simulink model "mnist_cnn_adam_figure"  (R2017b)
settings: Solver=FixedStepDiscrete  StartTime=0.0  StopTime=Inf  FixedStep=1  RelTol=1e-3
model workspace (MATLAB code in the model file):
  | filtersize1 = 5;
  | filtersize2 = 5;
  | features1 = 16;
  | features2 = 16;
  | densesize = 64;
  | classes = 10;
  | batchsize = 64;
libraries: ad_blocks x24
settings Model: PauseTimes=2  SnapshotBufferSize=2  SnapshotInterval=1  Creator=percro2  LastModifiedBy=eruffaldi
settings DataIOCC: ReturnWorkspaceOutputs=on
settings OptimizationCC: DefaultParameterBehavior=Inlined  InlineInvariantSignals=on  SimCompilerOptimization=on
settings RTWCC: GenerateReport=on  Toolchain=Clang v3.1 | gmake (64-bit Mac)  BuildConfiguration=Specify  LaunchReport=on
settings CodeAppCC: StateflowObjectComments=on  MATLABSourceComments=on
settings GRTTargetCC: CodeReplacementLibrary=GNU C99 extensions

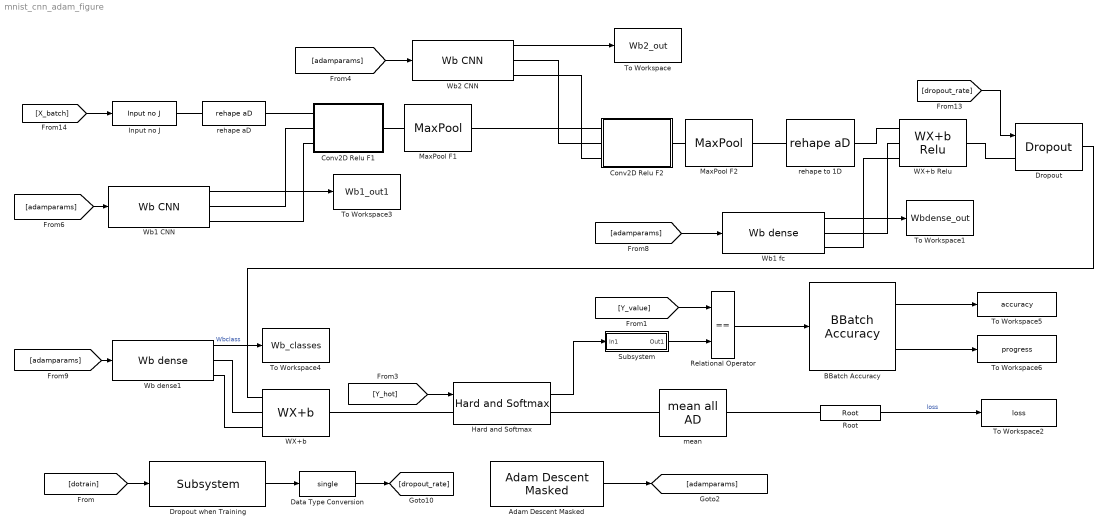
== system mnist_cnn_adam_figure ==
  Adam Descent Masked : ad_blocks/Adam Descent Masked  learningrate=1e-4  beta1=0.9  beta2=0.9999  epsilon=1e-8  adam=on
  BBatch Accuracy : ad_blocks/BBatch Accuracy
  Conv2D Relu F1 : Subsystem
  Conv2D Relu F2 : Subsystem
  Data Type Conversion : DataTypeConversion  OutDataTypeStr=single
  Dropout : ad_blocks/Dropout
  Dropout when Training : ad_blocks/Subsystem  dropout_rate=0.8
  Hard and Softmax : ad_blocks/Hard and Softmax
  Input no J : ad_blocks/Input no J  SystemSampleTime=-1
  MaxPool F1 : ad_blocks/MaxPool  stride=[1,2,2,1]  ksize=[1,2,2,1]  padding=-1
  MaxPool F2 : ad_blocks/MaxPool  stride=[1,2,2,1]  ksize=[1,2,2,1]  padding=-1
  Relational Operator : RelationalOperator  Operator===  OutDataTypeStr=boolean  RndMeth=Simplest
  Root : ad_blocks/Root  Description=Top level AD block: gets the incoming value, pushes the scalar 1 gradient  SystemSampleTime=-1
  Subsystem : Subsystem
  To Workspace : ToWorkspace  VariableName=Wb2_out  SaveFormat=Timeseries  SampleTime=-1
      settings: MaxDataPoints=1
  To Workspace1 : ToWorkspace  VariableName=Wbdense_out  SaveFormat=Timeseries  SampleTime=-1
      settings: MaxDataPoints=1
  To Workspace2 : ToWorkspace  VariableName=loss  SaveFormat=Timeseries  SampleTime=-1
      settings: MaxDataPoints=1
  To Workspace3 : ToWorkspace  VariableName=Wb1_out1  SaveFormat=Timeseries  SampleTime=-1
      settings: MaxDataPoints=1
  To Workspace4 : ToWorkspace  VariableName=Wb_classes  SaveFormat=Timeseries  SampleTime=-1
      settings: MaxDataPoints=1
  To Workspace5 : ToWorkspace  VariableName=accuracy  SaveFormat=Timeseries  SampleTime=-1
      settings: MaxDataPoints=1
  To Workspace6 : ToWorkspace  VariableName=progress  SaveFormat=Timeseries  SampleTime=-1
      settings: MaxDataPoints=1
  "WX+b " : ad_blocks/WX+b 
  WX+b Relu : ad_blocks/WX+b Relu
  Wb dense1 : ad_blocks/Wb dense  wshape=[densesize,classes]
  Wb1 CNN : ad_blocks/Wb CNN  K=filtersize1  Fi=1  Fo=features1
  Wb1 fc : ad_blocks/Wb dense  wshape=[7*7*features2,densesize]
  Wb2 CNN : ad_blocks/Wb CNN  K=filtersize2  Fi=features1  Fo=features2
  mean : ad_blocks/mean all AD
  rehape aD : ad_blocks/rehape aD  shape=[-1,28,28]
  rehape to 1D : ad_blocks/rehape aD  shape=[-1,-1]
  wires:
  [Y_value] -> Relational Operator/1
  Wb2 CNN/1 -> To Workspace/1
  [adamparams] -> Wb2 CNN/1
  [adamparams] -> Wb1 CNN/1
  Wb1 CNN/1 -> To Workspace3/1
  Wb1 fc/1 -> To Workspace1/1
  [adamparams] -> Wb1 fc/1
  Wb dense1/1 -> To Workspace4/1  "Wbclass"
  [adamparams] -> Wb dense1/1
  Relational Operator/1 -> BBatch Accuracy/2
  Dropout when Training/1 -> Data Type Conversion/1
  [dropout_rate] -> Dropout/1
  [dotrain] -> Dropout when Training/1
  Data Type Conversion/1 -> [dropout_rate]
  [X_batch] -> Input no J/1
  BBatch Accuracy/1 -> To Workspace5/1
  Root/1 -> To Workspace2/1  "loss"
  [Y_hot] -> Hard and Softmax/1
  Hard and Softmax/1 -> Subsystem/1(In1)
  Adam Descent Masked/1 -> [adamparams]
  Subsystem/1(Out1) -> Relational Operator/2
  BBatch Accuracy/2 -> To Workspace6/1
  connections:
  rehape aD/LConn1 -- Input no J/RConn1
  mean/RConn1 -- Root/LConn1
  MaxPool F2/LConn1 -- Conv2D Relu F2/RConn1
  rehape to 1D/LConn1 -- MaxPool F2/RConn1
  Dropout/LConn1 -- WX+b Relu/RConn1
  "WX+b "/LConn1 -- Dropout/RConn1
  "WX+b "/LConn2 -- Wb dense1/RConn1
  "WX+b "/LConn3 -- Wb dense1/RConn2
  Wb1 CNN/RConn2 -- Conv2D Relu F1/LConn3
  rehape to 1D/RConn1 -- WX+b Relu/LConn1
  Wb2 CNN/RConn1 -- Conv2D Relu F2/LConn2
  Wb2 CNN/RConn2 -- Conv2D Relu F2/LConn3
  Wb1 fc/RConn1 -- WX+b Relu/LConn2
  Wb1 fc/RConn2 -- WX+b Relu/LConn3
  Hard and Softmax/LConn1 -- "WX+b "/RConn1
  Hard and Softmax/RConn1 -- mean/LConn1
  MaxPool F1/RConn1 -- Conv2D Relu F2/LConn1
  Conv2D Relu F1/RConn1 -- MaxPool F1/LConn1
  rehape aD/RConn1 -- Conv2D Relu F1/LConn1
  Wb1 CNN/RConn1 -- Conv2D Relu F1/LConn2

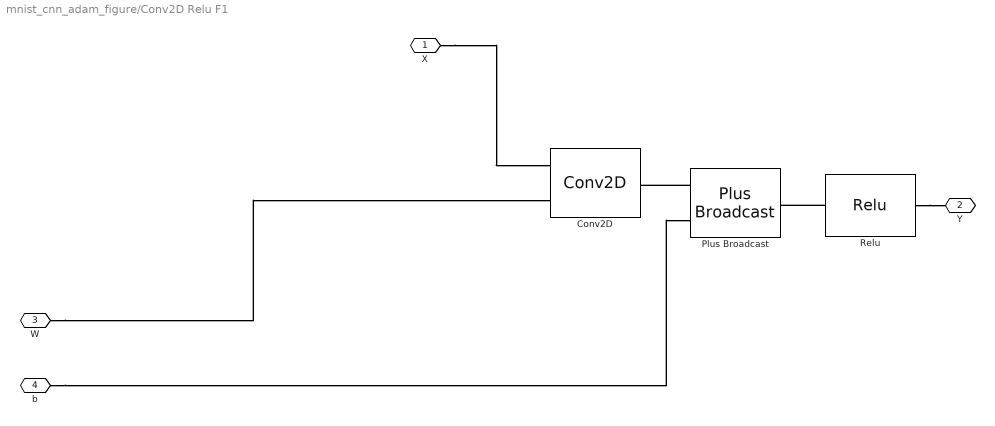
== system mnist_cnn_adam_figure/Conv2D Relu F1 ==
  Conv2D : ad_blocks/Conv2D  stride=[1,1,1,1]  padding=-1
  Plus Broadcast : ad_blocks/Plus Broadcast
  Relu : ad_blocks/Relu
  X : PMIOPort  Port=1  Side=Left
  Y : PMIOPort  Port=2  Side=Right
  W : PMIOPort  Port=3  Side=Left
  b : PMIOPort  Port=4  Side=Left
  connections:
  Relu/LConn1 -- Plus Broadcast/RConn1
  Plus Broadcast/LConn1 -- Conv2D/RConn1
  Relu/RConn1 -- Y/RConn1
  b/RConn1 -- Plus Broadcast/LConn2
  X/RConn1 -- Conv2D/LConn1
  W/RConn1 -- Conv2D/LConn2

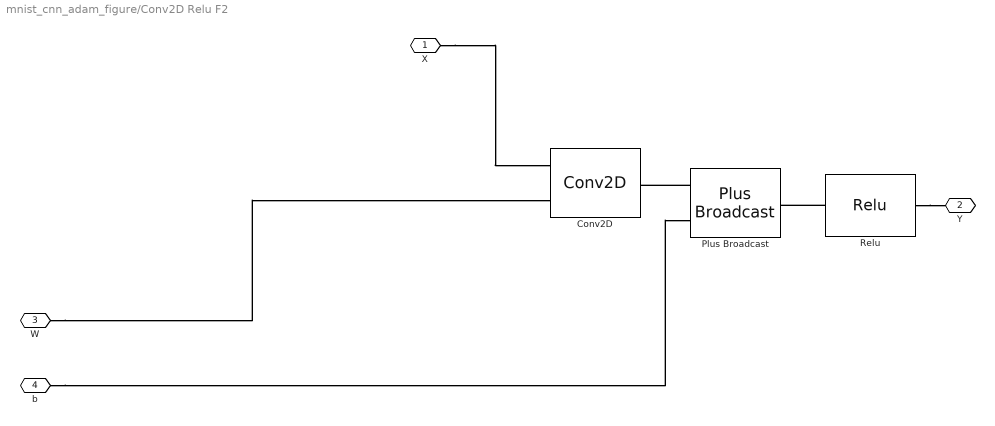
== system mnist_cnn_adam_figure/Conv2D Relu F2 ==
  Conv2D : ad_blocks/Conv2D  stride=[1,1,1,1]  padding=-1
  Plus Broadcast : ad_blocks/Plus Broadcast
  Relu : ad_blocks/Relu
  X : PMIOPort  Port=1  Side=Left
  Y : PMIOPort  Port=2  Side=Right
  W : PMIOPort  Port=3  Side=Left
  b : PMIOPort  Port=4  Side=Left
  connections:
  W/RConn1 -- Conv2D/LConn2
  X/RConn1 -- Conv2D/LConn1
  b/RConn1 -- Plus Broadcast/LConn2
  Relu/RConn1 -- Y/RConn1
  Plus Broadcast/LConn1 -- Conv2D/RConn1
  Relu/LConn1 -- Plus Broadcast/RConn1

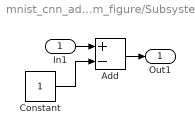
== system mnist_cnn_adam_figure/Subsystem ==
  In1 : Inport
  Add : Sum  Inputs=+-
  Constant : Constant  OutDataTypeStr=Inherit: Inherit via back propagation
  Out1 : Outport
  wires:
  In1/1 -> Add/1
  Add/1 -> Out1/1
  Constant/1 -> Add/2
